simulink model "lab12sim"  (R2020a)
settings: Solver=VariableStepAuto  StartTime=0.0  StopTime=30  RelTol=1e-3
settings Model: Creator=ariana  LastModifiedBy=ariana

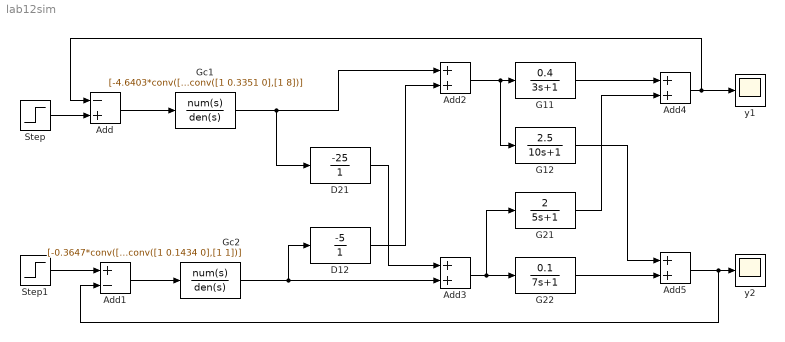
== system lab12sim ==
  Add : Sum  Inputs=-+
  Add1 : Sum  Inputs=+-
  Add{2..5} (4 alike) : Sum
  D12 : TransferFcn  Numerator=[-5]  Denominator=[1]
  D21 : TransferFcn  Numerator=[-25]  Denominator=[1]
  G11 : TransferFcn  Numerator=[0.4]  Denominator=[3 1]
  G12 : TransferFcn  Numerator=[2.5]  Denominator=[10 1]
  G21 : TransferFcn  Numerator=[2]  Denominator=[5 1]
  G22 : TransferFcn  Numerator=[0.1]  Denominator=[7 1]
  Gc1 : TransferFcn  Numerator=[-4.6403*conv([1 0.3333],[1 0.2])]  Denominator=[conv([1 0.3351 0],[1 8])]
  Gc2 : TransferFcn  Numerator=[-0.3647*conv([1 0.1429],[1 0.1])]  Denominator=[conv([1 0.1434 0],[1 1])]
  Step : Step  Time=0  SampleTime=0
  Step1 : Step  Time=0  SampleTime=0
  y1 : Scope
  y2 : Scope
  wires:
  Add/1 -> Gc1/1
  Add1/1 -> Gc2/1
  Gc1/1 -> D21/1, Add2/1
  D12/1 -> Add2/2
  Gc2/1 -> Add3/2, D12/1
  D21/1 -> Add3/1
  Add2/1 -> G12/1, G11/1
  Add3/1 -> G21/1, G22/1
  G22/1 -> Add5/2
  G11/1 -> Add4/1
  G12/1 -> Add5/1
  G21/1 -> Add4/2
  Add4/1 -> Add/1, y1/1
  Add5/1 -> Add1/2, y2/1
  Step/1 -> Add/2
  Step1/1 -> Add1/1
